simulink model "massSpringDamper"  (R2025b)
settings: Solver=VariableStepAuto  StartTime=0.0  StopTime=10.0  RelTol=1e-3
settings Model: Creator=lando  LastModifiedBy=lando

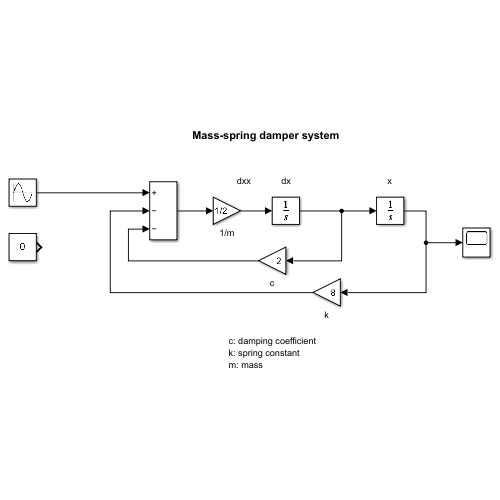
[thumbnail: Simulink's stored preview of the top-level diagram]
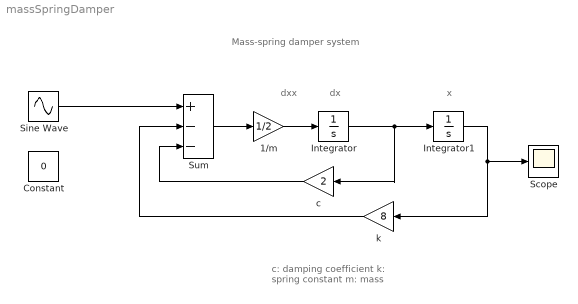
== system massSpringDamper ==
  note: c: damping coefficient
      | k: spring constant
      | m: mass
  note: x
  note: dxx
  note: Mass-spring damper system
  note: dx
  1/m : Gain  Gain=1/2
  Constant : Constant  Value=0
  Integrator : Integrator  InitialCondition=5
  Integrator1 : Integrator  InitialCondition=1
  Scope : Scope
      settings: ActiveDisplayYMinimum=-7.7581691085876345  ActiveDisplayYMaximum=6.130193849466905
  Sine Wave : Sin  Amplitude=2  Frequency=2  SampleTime=0
  Sum : Sum  Inputs=+--
  c : Gain  Gain=2
  k : Gain  Gain=8
  wires:
  Integrator/1 -> c/1, Integrator1/1
  Integrator1/1 -> k/1, Scope/1
  Sum/1 -> 1/m/1
  Sine Wave/1 -> Sum/1
  k/1 -> Sum/2
  c/1 -> Sum/3
  1/m/1 -> Integrator/1
